simulink model "Wider_System"  (R2023a)
settings: Solver=FixedStepDiscrete  StartTime=0.0  StopTime=20  FixedStep=0.01  RelTol=1e-3
libraries: SignalEditorBlockLib x1, simulink x1
settings Model: Creator=gaming3  LastModifiedBy=gaming3
settings OptimizationCC: DefaultParameterBehavior=Inlined  UseDivisionForNetSlopeComputation=on  GainParamInheritBuiltInType=on  UseFloatMulNetSlope=on  InlineInvariantSignals=on  PassReuseOutputArgsAs=Individual arguments  ZeroExternalMemoryAtStartup=off  ZeroInternalMemoryAtStartup=off  NoFixptDivByZeroProtection=on  EfficientFloat2IntCast=on  LifeSpan=1  OptimizeBlockOrder=speed  DifferentSizesBufferReuse=on  EfficientTunableParamExpr=on
settings DebuggingCC: ParameterTunabilityLossMsg=error
settings HardwareCC: ProdBitPerInt=16  ProdBitPerPointer=8  ProdBitPerSizeT=24  ProdBitPerPtrDiffT=24  ProdLargestAtomicFloat=None  ProdWordSize=8  ProdLongLongMode=on  ProdHWDeviceType=Microchip->PIC18
settings SFSimCC: MATLABDynamicMemAlloc=off
settings RTWCC: Description=Embedded Coder  SystemTargetFile=ert.tlc  GenCodeOnly=on  TemplateMakefile=ert_default_tmf
settings CodeAppCC: ForceParamTrailComments=on  IgnoreCustomStorageClasses=off  OperatorAnnotations=on  SimulinkDataObjDesc=on  SFDataObjDesc=on  CustomSymbolStrGlobalVar=rt$N$M  CustomSymbolStrType=$N$M  CustomSymbolStrFcn=$N$M$F  CustomSymbolStrMacro=$N$M  InsertBlockDesc=on
settings ERTTargetCC: TargetLangStandard=C99 (ISO)  GenerateSampleERTMain=on  IncludeMdlTerminateFcn=off  CombineSignalStateStructs=on  SupportComplex=off  SupportContinuousTime=on  SupportNonInlinedSFcns=on  InlinedParameterPlacement=NonHierarchical  ERTCustomFileTemplate=example_file_process.tlc  ERTFilePackagingFormat=CompactWithDataFile

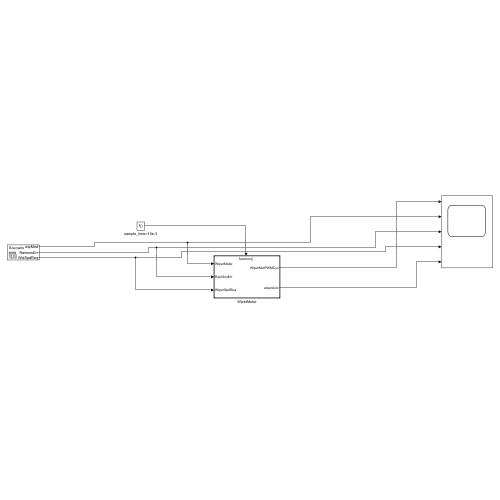
[thumbnail: Simulink's stored preview of the top-level diagram]
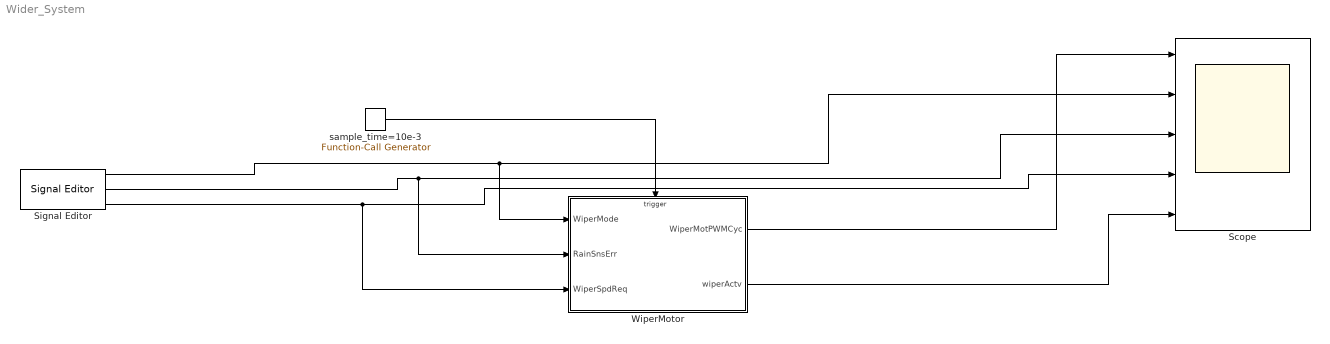
== system Wider_System ==
  Scope : Scope  NumInputPorts=5
  Signal Editor : SignalEditorBlockLib/Signal Editor  FileName=D:\work\MBD\projects\signals\widerMotor.mat  ActiveScenario=Scenario  ActiveSignal=wipMod  IsBus=off  OutputBusObjectStr=Bus: BusObject  SampleTime=0  ZeroCross=off  OutputAfterFinalValue=Setting to zero  Unit=inherit  PreserveSignalName=on  ApplySigPropsToAllScenarios=on
  WiperMotor : Subsystem  TreatAsAtomicUnit=on
  sample_time=10e-3 : simulink/Ports & Subsystems/Function-Call Generator  sample_time=0.01  numberOfIterations=1  DisallowWideOutput=off
  wires:
  WiperMotor/1(WiperMotPWMCyc) -> Scope/1
  WiperMotor/2(wiperActv) -> Scope/5
  sample_time=10e-3/1 -> WiperMotor/Trigger
  Signal Editor/3 -> WiperMotor/3(WiperSpdReq), Scope/4
  Signal Editor/1 -> WiperMotor/1(WiperMode), Scope/2
  Signal Editor/2 -> WiperMotor/2(RainSnsErr), Scope/3

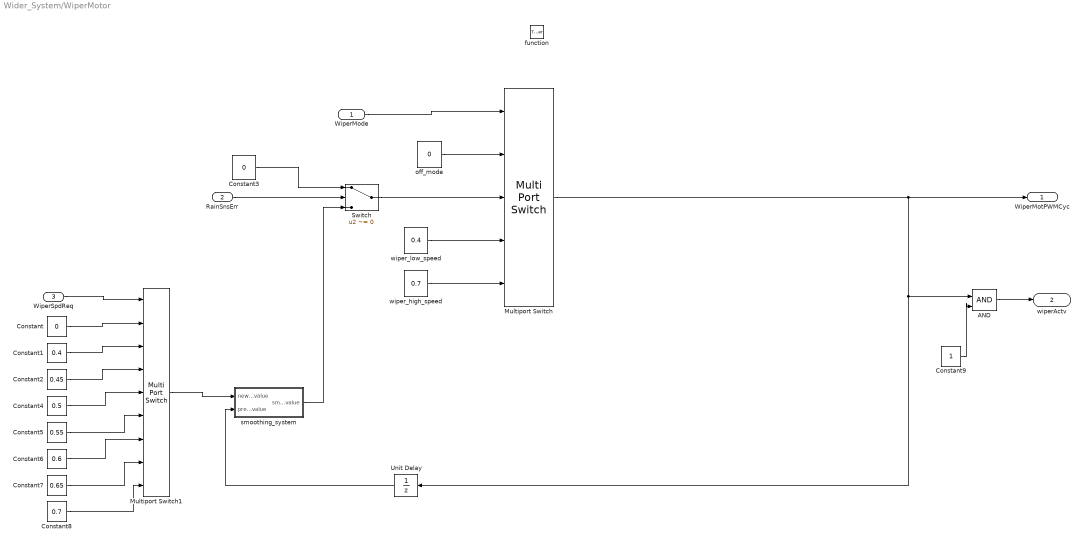
== system Wider_System/WiperMotor ==
  WiperMode : Inport
  RainSnsErr : Inport  Port=2  OutDataTypeStr=boolean
  WiperSpdReq : Inport  Port=3
  function : TriggerPort  TriggerType=function-call  VariantControl=(inherit)
  AND : Logic  IconShape=distinctive  AllPortsSameDT=off  OutDataTypeStr=boolean
  Constant : Constant  Value=0
  Constant1 : Constant  Value=0.4
  Constant2 : Constant  Value=0.45
  Constant3 : Constant  Value=0
  Constant4 : Constant  Value=0.5
  Constant5 : Constant  Value=0.55
  Constant6 : Constant  Value=0.6
  Constant7 : Constant  Value=0.65
  Constant8 : Constant  Value=0.7
  Constant9 : Constant
  Multiport Switch : MultiPortSwitch  DataPortOrder=Zero-based contiguous  Inputs=4  zeroidx=on  SaturateOnIntegerOverflow=off  InputSameDT=off
  Multiport Switch1 : MultiPortSwitch  DataPortOrder=Zero-based contiguous  Inputs=8  zeroidx=on  SaturateOnIntegerOverflow=off  InputSameDT=off
  Switch : Switch  Criteria=u2 ~= 0  SaturateOnIntegerOverflow=off  InputSameDT=off
  Unit Delay : UnitDelay  SampleTime=-1  HasFrameUpgradeWarning=on
  off_mode : Constant  Value=0
  smoothing_system : Subsystem
  wiper_high_speed : Constant  Value=0.7
  wiper_low_speed : Constant  Value=0.4
  WiperMotPWMCyc : Outport
  wiperActv : Outport  Port=2
  wires:
  Constant5/1 -> Multiport Switch1/6
  Constant9/1 -> AND/2
  Multiport Switch1/1 -> smoothing_system/1(new_value)
  Constant3/1 -> Switch/1
  smoothing_system/1(smoothed_value) -> Switch/3
  AND/1 -> wiperActv/1
  Constant4/1 -> Multiport Switch1/5
  Constant7/1 -> Multiport Switch1/8
  Switch/1 -> Multiport Switch/3
  WiperSpdReq/1 -> Multiport Switch1/1
  Constant/1 -> Multiport Switch1/2
  Unit Delay/1 -> smoothing_system/2(prev_value)
  WiperMode/1 -> Multiport Switch/1
  wiper_high_speed/1 -> Multiport Switch/5
  wiper_low_speed/1 -> Multiport Switch/4
  Constant6/1 -> Multiport Switch1/7
  Constant1/1 -> Multiport Switch1/3
  Multiport Switch/1 -> WiperMotPWMCyc/1, Unit Delay/1, AND/1
  off_mode/1 -> Multiport Switch/2
  Constant2/1 -> Multiport Switch1/4
  Constant8/1 -> Multiport Switch1/9
  RainSnsErr/1 -> Switch/2

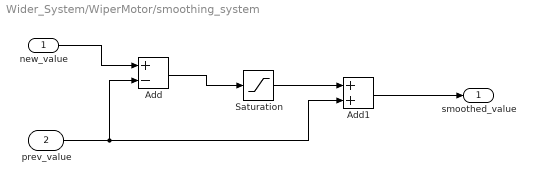
== system Wider_System/WiperMotor/smoothing_system ==
  new_value : Inport
  prev_value : Inport  Port=2
  Add : Sum  Inputs=+-
  Add1 : Sum
  Saturation : Saturate  UpperLimit=0.005  LowerLimit=-0.005
  smoothed_value : Outport
  wires:
  Add1/1 -> smoothed_value/1
  prev_value/1 -> Add/2, Add1/2
  Saturation/1 -> Add1/1
  Add/1 -> Saturation/1
  new_value/1 -> Add/1
